simulink model "adcs_v11_log"  (Simulink 7.4)
settings: Solver=ode4  StartTime=0.0  StopTime=80000  FixedStep=s_SIM_STEP_SIZE  RelTol=1e-3
values from neighbouring files (symbols this model uses):
  A = ((T_SIDE + .29)*1e-3)^2    [constants_v13.m]    (also in constants_v15.m; constants_v15_Pow.m; constants_v15_Pow_ss_error.m; constants_v16_integral_kartavya.m)
  Ca_Solar_Drag = 1.4    [constants_v13.m]    (also in constants_v15.m; constants_v15_Pow.m; constants_v15_Pow_ss_error.m; constants_v16_integral_kartavya.m)
  Cd = 2.2    [constants_v13.m]    (also in constants_v15.m; constants_v15_Pow.m; constants_v15_Pow_ss_error.m; constants_v16_integral_kartavya.m)
  check_time = 60000    [constants_v13.m]    (also in constants_v15.m = 10000; constants_v15_Pow.m = 10000; constants_v15_Pow_ss_error.m = 10000; constants_v16_integral_kartavya.m = 10000)
  equinox = datenum('21-Mar-2010 12:0:0')    [constants_v13.m]    (also in constants_v15.m; constants_v15_Pow.m; constants_v15_Pow_ss_error.m; constants_v16_integral_kartavya.m)
  err_SGP = 0    [constants_v16_integral_kartavya.m]    (also in constants_v16_integral_light_sun_sgp_igrf_power_13Dec2011.m)
  I_MAX = 0.5    [constants_v13.m]    (also in constants_v15.m; constants_v15_Pow.m; constants_v15_Pow_ss_error.m; constants_v16_integral_kartavya.m)
  I_TORQUER = 3.6 / 7.31    (= 0.492476060192)    [constants_v13.m]    (also in constants_v15.m; constants_v15_Pow.m; constants_v15_Pow_ss_error.m; constants_v16_integral_kartavya.m)
  Kd = 2* m_INERTIA / (s_numOrbits * T_ORBIT )    [constants_v13.m]    (also in constants_v15.m = m_INERTIA * (2 + delta)* zeta * w; constants_v15_Pow.m = m_INERTIA * (2 + delta)* zeta * w; constants_v15_Pow_ss_error.m = m_INERTIA * (2 + delta)* zeta * w; constants_v16_integral_kartavya.m = m_INERTIA * (2 + delta)* zeta * w)
  Kdetumb = K_det*eye(3)    [constants_v13.m]    (also in constants_v15.m; constants_v15_Pow.m; constants_v15_Pow_ss_error.m; constants_v16_integral_kartavya.m)
  Kp = m_INERTIA / (s_numOrbits * T_ORBIT * zeta)^2    [constants_v13.m]    (also in constants_v15.m = m_INERTIA * (w*w + 2*delta*zeta^2*w^2); constants_v15_Pow.m = m_INERTIA * (w*w + 2*delta*zeta^2*w^2); constants_v15_Pow_ss_error.m = m_INERTIA * (w*w + 2*delta*zeta^2*w^2); constants_v16_integral_kartavya.m = m_INERTIA * (w*w + 2*delta*zeta^2*w^2))
  m_INERTIA = [Ixx Ixy Ixz; Ixy Iyy Iyz; Ixz Iyz Izz]    [constants_v13.m]    (also in constants_v15.m; constants_v15_Pow.m = 1*[Ixx Ixy Ixz; Ixy Iyy Iyz; Ixz Iyz Izz]; constants_v15_Pow_ss_error.m = 1*[Ixx Ixy Ixz; Ixy Iyy Iyz; Ixz Iyz Izz]; constants_v16_integral_kartavya.m)
  mu = 6.673e-11*5.9742e24    (= 398658366000000)    [constants_v13.m]    (also in constants_v15.m; constants_v15_Pow.m; constants_v15_Pow_ss_error.m; constants_v16_integral_kartavya.m)
  N = 40    [constants_v13.m]    (also in constants_v15.m; constants_v15_Pow.m; constants_v15_Pow_ss_error.m; constants_v16_integral_kartavya.m)
  P_momentum_flux_from_the_sun = 4.4e-6    (= 4.4e-06)    [constants_v13.m]    (also in constants_v15.m; constants_v15_Pow.m; constants_v15_Pow_ss_error.m; constants_v16_integral_kartavya.m)
  q_BI0 = euler2qBI(roll0,pitch0,yaw0)    [constants_v13.m]    (also in constants_v15.m; constants_v15_Pow.m; constants_v15_Pow_ss_error.m; constants_v16_integral_kartavya.m)
  s_AU = 159597870610    [constants_v16_integral_kartavya.m]    (also in constants_v16_integral_light_sun_sgp_igrf_power_13Dec2011.m; light_calc.m)
  s_DOY = sime(2)*30 - 30 + sime(3)    [constants_v16_integral_kartavya.m]    (also in constants_v16_integral_light_sun_sgp_igrf_power_13Dec2011.m; precalcs.m)
  s_FRAME_SIZE = 2    [constants_v13.m]    (also in constants_v15.m; constants_v15_Pow.m; constants_v15_Pow_ss_error.m; constants_v16_integral_kartavya.m)
  s_m_MAX = 0.95    [constants_v13.m]    (also in constants_v15.m; constants_v15_Pow.m; constants_v15_Pow_ss_error.m; constants_v16_integral_kartavya.m)
  s_MAG_B = 2.5e-5    (= 2.5e-05)    [constants_v13.m]    (also in constants_v15.m; constants_v15_Pow.m; constants_v15_Pow_ss_error.m; constants_v16_integral_kartavya.m)
  s_MAGMETER_WEIGHT = .9    (= 0.9)    [constants_v13.m]    (also in constants_v15.m; constants_v15_Pow.m; constants_v15_Pow_ss_error.m; constants_v16_integral_kartavya.m)
  s_Rearth = 6378164    [constants_v16_integral_kartavya.m]    (also in constants_v16_integral_light_sun_sgp_igrf_power_13Dec2011.m; light_calc.m)
  s_Rsun = 695500000    [constants_v16_integral_kartavya.m]    (also in constants_v16_integral_light_sun_sgp_igrf_power_13Dec2011.m; light_calc.m)
  s_SEC = sime(4)*3600 + sime(5)*60 + sime(6)    [constants_v16_integral_kartavya.m]    (also in constants_v16_integral_light_sun_sgp_igrf_power_13Dec2011.m; precalcs.m)
  s_SIM_STEP_SIZE = 0.1    [constants_v13.m]    (also in constants_v15.m; constants_v15_Pow.m; constants_v15_Pow_ss_error.m; constants_v16_integral_kartavya.m)
  s_SS_ADC_gain = 5    [constants_v13.m]    (also in constants_v15.m; constants_v15_Pow.m; constants_v15_Pow_ss_error.m; constants_v16_integral_kartavya.m)
  s_SS_ADC_res = 2^12 - 1    (= 4095)    [constants_v13.m]    (also in constants_v15.m; constants_v15_Pow.m; constants_v15_Pow_ss_error.m; constants_v16_integral_kartavya.m)
  s_SS_MAX_ANGLE = 85    [constants_v13.m]    (also in constants_v15.m; constants_v15_Pow.m; constants_v15_Pow_ss_error.m; constants_v16_integral_kartavya.m)
  s_W_SAT = sqrt(mu/R_e^3)    [constants_v13.m]    (also in constants_v15.m; constants_v15_Pow.m; constants_v15_Pow_ss_error.m; constants_v16_integral_kartavya.m)
  s_x_MAGMETER_BIAS = 50e-9    (= 5e-08)    [constants_v13.m]    (also in constants_v15.m; constants_v15_Pow.m; constants_v15_Pow_ss_error.m; constants_v16_integral_kartavya.m)
  s_YEAR = sime(1) + (sime(2)*30 - 30 + sime(3))/365    [constants_v16_integral_kartavya.m]    (also in constants_v16_integral_light_sun_sgp_igrf_power_13Dec2011.m; precalcs.m)
  side = 0.26    [constants_v13.m]    (also in constants_v15.m; constants_v15_Pow.m; constants_v15_Pow_ss_error.m; constants_v16_integral_kartavya.m)
  Snum = 6    [constants_v13.m]    (also in constants_v15.m; constants_v15_Pow.m; constants_v15_Pow_ss_error.m; constants_v16_integral_kartavya.m)
  stperut = 1.00273790935    [constants_v16_integral_kartavya.m]    (also in constants_v16_integral_light_sun_sgp_igrf_power_13Dec2011.m; precalcs.m)
  t_reset = 600    [constants_v16_integral_kartavya.m]    (also in constants_v16_integral_light_sun_sgp_igrf_power_13Dec2011.m; precalcs.m)
  TLE_epoch = datenum('18-Oct-2010 10:30:0')    [constants_v16_integral_kartavya.m]    (also in constants_v16_integral_light_sun_sgp_igrf_power_13Dec2011.m; precalcs.m)
  today = datenum('18-Oct-2010 10:30:0')    [constants_v13.m]    (also in constants_v15.m; constants_v15_Pow.m; constants_v15_Pow_ss_error.m; constants_v16_integral_kartavya.m)
  tol_w = 4e-3    (= 0.004)    [constants_v13.m]    (also in constants_v15.m; constants_v15_Pow.m; constants_v15_Pow_ss_error.m; constants_v16_integral_kartavya.m)
  Ts_display = 6    [constants_v13.m]    (also in constants_v15.m; constants_v15_Pow.m; constants_v15_Pow_ss_error.m; constants_v16_integral_kartavya.m)
  v_COM_to_COP_b = [.2; 1.75; .2]*1e-2    [constants_v13.m]    (also in constants_v15.m; constants_v15_Pow.m; constants_v15_Pow_ss_error.m; constants_v16_integral_kartavya.m)
  v_S1 = [1 0 0]    [constants_v13.m]    (also in constants_v15.m; constants_v15_Pow.m; constants_v15_Pow_ss_error.m; constants_v16_integral_kartavya.m)
  v_S2 = [-1 0 0]    [constants_v13.m]    (also in constants_v15.m; constants_v15_Pow.m; constants_v15_Pow_ss_error.m; constants_v16_integral_kartavya.m)
  v_S3 = [0 1 0]    [constants_v13.m]    (also in constants_v15.m; constants_v15_Pow.m; constants_v15_Pow_ss_error.m; constants_v16_integral_kartavya.m)
  v_S4 = [0 -1 0]    [constants_v13.m]    (also in constants_v15.m; constants_v15_Pow.m; constants_v15_Pow_ss_error.m; constants_v16_integral_kartavya.m)
  v_S5 = [0 0 1]    [constants_v13.m]    (also in constants_v15.m; constants_v15_Pow.m; constants_v15_Pow_ss_error.m; constants_v16_integral_kartavya.m)
  v_S6 = [0 0 -1]    [constants_v13.m]    (also in constants_v15.m; constants_v15_Pow.m; constants_v15_Pow_ss_error.m; constants_v16_integral_kartavya.m)
  v_x_MOUNTING_THETA_ZYX_BODY_TORQUER = [1; 1; 1]* pi/180    [constants_v13.m]    (also in constants_v15.m; constants_v15_Pow.m; constants_v15_Pow_ss_error.m; constants_v16_integral_kartavya.m)
  W_EARTH_ROT = 2*pi/86400    (= 7.27220521664e-05)    [constants_v16_integral_kartavya.m]    (also in constants_v16_integral_light_sun_sgp_igrf_power_13Dec2011.m; precalcs.m)
  wx0 = 2*pi/180    (= 0.0349065850399)    [constants_v13.m]    (also in constants_v15.m = 0.00174532925199; constants_v15_Pow.m = 1.74532925199e-05; constants_v15_Pow_ss_error.m = 2.01533262693e-05; constants_v16_integral_kartavya.m = 0.0174532925199)
  wy0 = 1*pi/180    (= 0.0174532925199)    [constants_v13.m]    (also in constants_v15.m = 0.00174532925199; constants_v15_Pow.m = 1.74532925199e-05; constants_v15_Pow_ss_error.m = 2.01533262693e-05; constants_v16_integral_kartavya.m = 0)
  wz0 = -2*pi/180    (= -0.0349065850399)    [constants_v13.m]    (also in constants_v15.m = 0.00174532925199; constants_v15_Pow.m = 1.74532925199e-05; constants_v15_Pow_ss_error.m = 2.01533262693e-05; constants_v16_integral_kartavya.m = -0.00872664625997)
undefined symbols (not defined in the file or in its folder): Earth, s_omega_MAX, s_YEAR_ONLY, tol_pitch, tol_roll, tol_yaw, v_S10, v_S11, v_S12, v_S7, v_S8, v_S9, v_Si0, WGS84
libraries: commnoisgen2 x15, aerolibutil x7, aerolibtransform2 x5, dspsigops x5, powerlib_extras x3, aerolibgravity2 x2, aerolibatmos2 x1, dspmtrx3 x1, simulink x1
(part 3 of 3)

== matlab function Embedded MATLAB Function4 ==
  data: euler output double; v_Si input double; x input double; q_BO output double; w_BOB output double; modw output double; s_W_SAT parameter double; w_BIB output double
function [euler, q_BO, w_BOB, modw, w_BIB] = qBO(v_Si, x, s_W_SAT)
% This block supports the Embedded MATLAB subset.
% See the help menu for details. 

% ECI to TIO 
r = v_Si(1:3);   % position vector in ECI
v = v_Si(4:6);   % velocity vector in ECI

oy = cross(v,r);    % orbit frame x...
oy = oy/sqrt(dot(oy,oy));

oz = -r/sqrt(dot(r,r));

ox = cross(oy,oz);
ox = ox/sqrt(dot(ox,ox));

TIO = [ox oy oz];

% qIO from TIO
if (trace(TIO) == -1)
    if ( TIO(1,2) == 0 && TIO(1,3) ==0 )
        q_IO = [1; 0; 0; 0];
    elseif ( TIO(1,2) == 0 && TIO(2,3) ==0 )
        q_IO = [0; 1; 0; 0];
    elseif ( TIO(1,3) == 0 && TIO(2,3) ==0 )
        q_IO = [0; 0; 1; 0];
    else
        e1 = TIO(1,2)*TIO(1,3);
        e2 = TIO(1,2)*TIO(2,3);
        e3 = TIO(1,3)*TIO(2,3);
        norm = sqrt( e1*e1 + e2*e2 + e3*e3);
        q_IO = [e1; e2; e3; 0]/norm;
    end        
else
    q4 = 0.5*sqrt(1 + trace(TIO));
    q1 = -(TIO(3,2) - TIO(2,3)) / (4*q4);
    q2 = -(TIO(1,3) - TIO(3,1)) / (4*q4);
    q3 = -(TIO(2,1) - TIO(1,2)) / (4*q4);
    q_IO = [q1; q2; q3; q4];
end

q_BI = x(1:4);

% q_BO = q_BI*q_IO
q_BIx = ...
[ q_BI(4)  q_BI(3) -q_BI(2) q_BI(1);
 -q_BI(3)  q_BI(4)  q_BI(1) q_BI(2);
  q_BI(2) -q_BI(1)  q_BI(4) q_BI(3);
 -q_BI(1) -q_BI(2) -q_BI(3) q_BI(4)];

q_BO = q_BIx * q_IO;

euler =  (180/pi)*[atan2( 2*( q_BO(4)*q_BO(1)-q_BO(2)*q_BO(3) ),( 1 - 2*( q_BO(1)^2 + q_BO(2)^2 ) )  ) ;
              asin( 2*(q_BO(4)*q_BO(2)+q_BO(3)*q_BO(1)) );
             atan2( 2*( q_BO(4)*q_BO(3)-q_BO(1)*q_BO(2) ),( 1 - 2*( q_BO(2)^2 + q_BO(3)^2 ) )  ) ];
         
w_BIB = x(5:7);
w_OIO = [0; -s_W_SAT; 0];

q0 = q_BO(4); q1 = q_BO(1); q2 = q_BO(2); q3 = q_BO(3);

TBO = [ q0^2 + q1^2 - q2^2 - q3^2,         2*q0*q3 + 2*q1*q2,         2*q1*q3 - 2*q0*q2;
           2*q1*q2 - 2*q0*q3, q0^2 - q1^2 + q2^2 - q3^2,         2*q0*q1 + 2*q2*q3;
           2*q0*q2 + 2*q1*q3,         2*q2*q3 - 2*q0*q1, q0^2 - q1^2 - q2^2 + q3^2];
       
w_OIB = TBO*w_OIO;
w_BOB = w_BIB - w_OIB;

modw = sqrt(dot(w_BOB,w_BOB));

== matlab function SGP /Subsystem/Embedded MATLAB Function1 ==
  data: TLE input double; modTLE output double
function modTLE  = convertTLE(TLE)
meanMo = TLE(19);
orbEcc = TLE(16);
orbInc = TLE(14);
meanAno = TLE(18);
argPer = TLE(17);
rghtAsc = TLE(15);
SGPdragp1 = TLE(8);
SGPdragp2 = TLE(9);
SGP4dragp = TLE(10);
EpYear = TLE(5);
EpJD = TLE(6);
EpTime = TLE(7);
revNo = TLE(20);
n0 = 2*pi*meanMo/1440; % Mean motion (rad/min)
e0 = orbEcc; % Eccentricity (0.0<=e0>=1.0)
i0 = pi*orbInc/180; % Inclination (rad)
M0 = pi*meanAno/180; % Mean anomaly (rad)
w0 = pi*argPer/180; % Argument of perigee (rad)
Ohm0 = pi*rghtAsc/180; % Right ascension of the ascending node (rad)
dn0 = 2*2*pi*SGPdragp1/(1440^2); % Rirst time derivative of mean motion(rad/min^2)
ddn0 = 6*2*pi*SGPdragp2/(1440^3); % Second time derivative of mean motion (rad/min^3)
Bstar = SGP4dragp; % SGP4 type drag coefficient
% Mean year (400 year period) in days:
meanYearDays = (400*365 + 4 * (100/4 - 1) + 1) / 400;
% Time of epoch (since y2k)
t0 = (EpYear*meanYearDays + EpJD + EpTime)*1440;
modTLE = [t0 dn0 ddn0 Bstar i0 Ohm0 e0 w0 M0 n0 revNo];

== matlab function SGP /Subsystem/Embedded MATLAB Function2 ==
  data: modTLE input double; dT input double; R output double; dR output double
function [R,dR] = sgp(modTLE,dT)
%This code is a matlab implementation of the SGP Fortran code in the
% Startrack report #3.
%
% The matlab code was derived mainly by porting and editing the
% FORTRAN routines in NORAD’s Spacetrack report #3.
% According to a statement in that report, the document is free
% of copyrights and open to unlimited public distribution.
%
% This matlab code is distributed under the same conditions
%
%
% Created 15/10-2001 by
% Klaus Krogsgaard & Torsten Lorentzen
% - - - - - - - - - - - - - - - - - - - - - - - - -
%
% SGP model for predicting orbit position.
%

% - - - - - - - - - - - - - - - - - - - - - - - - -
% Constants given by the modified NORAD TLE (all at epoch)
% - - - - - - - - - - - - - - - - - - - - - - - - -


t0 = modTLE(1);
dn0 = modTLE(2); % first time derivative of the mean motion
ddn0 = modTLE(3); % second time derivative of mean motion
Bstar = modTLE(4); % Drag parameter
i0 = modTLE(5); % inclination
Ohm0 = modTLE(6); % right ascension of the ascending node
e0 = modTLE(7); % eccentricity
w0 = modTLE(8); % argument of perigee
M0 = modTLE(9); % mean anormaly
n0 = modTLE(10); % mean motion
revNo = modTLE(11); % Number of revolutions before epoch
% - - - - - - - - - - - - - - - - - - - - - - - - -
% Other constants
% - - - - - - - - - - - - - - - - - - - - - - - - -
GM = 398603 * 10^9;
er = 6378.135;
ke = 0.0743669161; %converted to er/min ^3/2
% aE = 6378160; % equatorial radius of the Earth
aE = 1;% give result in Earth radii
min_per_day = 1440;
sec_per_day = 86400;
km_per_er = er;
J2 = 5.413080*10^-4 * 2; % second gravitational zonal harmonic of the Earth
J3 = -0.253881*10^-5; % third gravitational zonal harmonic of the Earth
J4 = -0.62098875*10^-6 * 8/3; % fourth gravitational zonal harmonic of the Earth
% - - - - - - - - - - - - - - - - - - - - - - - - -
% Local constants
% - - - - - - - - - - - - - - - - - - - - - - - - -
a1 = (ke/n0)^(2/3);
delta1 = 3/4 * J2 * (aE/a1)^2 * (3*((cos(i0))^2)-1)/((1-e0^2)^(3/2));
a0 = a1 * (1 - 1/3*delta1 - delta1^2 - 134/81*delta1^3);
p0 = a0 * (1 - e0^2);
q0 = a0 * (1-e0);
L0 = M0 + w0 + Ohm0;
dOhm = - (3/2) * J2 * (aE/p0)^2 * n0 * cos(i0);
dw = (3/4) * J2 * (aE/p0)^2 * n0 * (5*(cos(i0))^2-1);
% - - - - - - - - - - - - - - - - - - - - - - - - -
% Secular effects of drag and gravitation
% - - - - - - - - - - - - - - - - - - - - - - - - -
a = a0 * ( n0 ./ (n0 + 2*(dn0/2)*(dT) + 3*(ddn0/6)*dT.^2)).^(2/3); % vector
e = zeros(1,length(dT)); % vector
for i=1:length(a)
if ( a(i)>q0 )
e(i) = 1 - q0/a(i);
else
e(i) = 10^-6;
end;
end;
p = a .* (1-e.^2); % vector
OhmS0 = Ohm0 + dOhm * dT; % vector
wS0 = w0 + dw * (dT); % vector
Ls = mod(L0 + (n0 + dw + dOhm)*(dT) + dn0/2 * (dT).^2 + ddn0/6 * (dT).^3,2*pi); % vector
% - - - - - - - - - - - - - - - - - - - - - - - - -
% Long period periodic effects
% - - - - - - - - - - - - - - - - - - - - - - - - -
axNSL = e .* cos(wS0); % vector
ayNSL = e .* sin(wS0) - 1/2 * J3/J2 * aE./p * sin(i0); % vector
L = mod(Ls - 1/4 * J3/J2 * aE./p .* axNSL * sin(i0) * (3+5*cos(i0))/(1+cos(i0)),2*pi); % vector
% - - - - - - - - - - - - - - - - - - - - - - - - -
% Iteration
% - - - - - - - - - - - - - - - - - - - - - - - - -
tol = 10^-8;
U = mod(L - OhmS0,2*pi); % vector
Ew1 = U; % vector
Ew2 = Ew1; % vector
dEw = (U - ayNSL.*cos(Ew1) + axNSL.*sin(Ew1) - Ew1) ./ (-ayNSL.*sin(Ew1) - axNSL.*cos(Ew1) + 1); % vector
for i=1:length(dEw)
if abs(dEw(i)) > 1
Ew2(i) = Ew1(i) + sign(dEw(i)); %vector
else
Ew2(i) = Ew1(i) + dEw(i);
end;
end;
for i=1:length(Ew1)
while abs(dEw(i))>tol
Ew1(i) = Ew2(i);
dEw(i) = (U(i) - ayNSL(i).*cos(Ew1(i)) + axNSL(i).*sin(Ew1(i)) - Ew1(i)) ./ ...
(-ayNSL(i).*sin(Ew1(i)) - axNSL(i).*cos(Ew1(i)) + 1);
if abs(dEw(i)) > 1
Ew2(i) = Ew1(i) + sign(dEw(i)); %vector
else
Ew2(i) = Ew1(i) + dEw(i);
end;
end;
end;
ecosE = axNSL.*cos(Ew2) + ayNSL.*sin(Ew2); % vector
esinE = axNSL.*sin(Ew2) - ayNSL.*cos(Ew2); % vector
SQeL = axNSL.^2 + ayNSL.^2; % vector
pL = a.*(1 - SQeL); % vector
r = a.*(1 - ecosE); % vector
dr = ke * sqrt(a)./r .* esinE; % vector
rdv = ke * sqrt(pL)./r; % vector
sinu = a./r .* (sin(Ew2) - ayNSL - axNSL.*esinE./(1+sqrt(1-SQeL))); % vector
cosu = a./r .* (cos(Ew2) - axNSL + ayNSL.*esinE./(1+sqrt(1-SQeL))); % vectro
u = mod(atan2( sinu,cosu ),2*pi); % vector
% - - - - - - - - - - - - - - - - - - - - - - - - -
% Short term perturbations
% - - - - - - - - - - - - - - - - - - - - - - - - -
rk = r + 1/4 * J2 * aE^2./pL * (sin(i0))^2 .* cos(2*u); % vector
uk = u - 1/8 * J2 * (aE./pL).^2 * (7 * (cos(i0))^2 - 1) .* sin(2*u); % vector
Ohmk = OhmS0 + 3/4 * J2 * (aE./pL).^2 * cos(i0) .* sin(2*u); % vector
ik = i0 + 3/4 * J2 * (aE./pL).^2 * sin(i0) * cos(i0) .* cos(2*u); % vector
% - - - - - - - - - - - - - - - - - - - - - - - - -
% Unit orientation vectors
% - - - - - - - - - - - - - - - - - - - - - - - - -
R = zeros(length(uk),3); % vector
dR = zeros(length(uk),3); % vector
for i=1:length(uk)
    M_vec = [ -sin(Ohmk(i))*cos(ik(i)) cos(Ohmk(i))*cos(ik(i)) sin(ik(i)) ]; % vector
N_vec = [ cos(Ohmk(i)) sin(Ohmk(i)) 0 ]; % vector
U_vec = M_vec * sin(uk(i)) + N_vec * cos(uk(i)); % vector
V_vec = M_vec * cos(uk(i)) - N_vec * sin(uk(i)); % vector
% - - - - - - - - - - - - - - - - - - - - - - - - -
% Position and velocity
% - - - - - - - - - - - - - - - - - - - - - - - - -
R(i,:) = rk(i) * U_vec; % vector
dR(i,:) = dr(i) * U_vec + rdv(i) * V_vec; % vector
end;
% - - - - - - - - - - - - - - - - - - - - - - - - -
% Transforming position to Cartesian coordinates in kilometers and velocity to kilometers/sec
% - - - - - - - - - - - - - - - - - - - - - - - - -
R = R * km_per_er /aE;
R = R * 1000; % km to m
dR = dR * km_per_er / aE * min_per_day / sec_per_day;
dR = dR * 1000; % km/s to m/s

== matlab function Sensors1/GPS/m_DCM_ECI-ECEF ==
  data: TEI output double; today input double; equinox input double; stperut input double; W_EARTH_ROT input double; t input double
function TEI = fcn(today,equinox, stperut,W_EARTH_ROT, t)
% This block gives DCM for converting from ECI to ECEF frames
% inputs: today's date, equinox, sidereal time per unit time, angular velocity of earth's rotation, simulation time
% output: DCM

% 23hr 56m 4.09s per day

ut_sec = (today - equinox)*24*60*60 + t; % universal time in sec
st_sec = stperut*ut_sec;    % sidereal time in sec

phi = st_sec*W_EARTH_ROT;            % sidereal time in rad

TEI = [ cos(phi) sin(phi) 0;
       -sin(phi) cos(phi) 0;
        0        0        1];
